simulink subsystem "AUVPlant"  (R2020a)
settings: Solver=VariableStepAuto  StartTime=0.0  StopTime=10.0  RelTol=1e-3
values from neighbouring files (symbols this model uses):
  N = [-39.9215617836 -39.7361560536 -39.4691718024 -38.8907059248 -38.267742672 -37.9562610456 -37.5112872936 -37.2888004176 -36.7993292904 -36.4433502888 -35.8648844112 -35.1974237832 ... (201 elements, 201x1)]    [matlab.mat]    (also in plant_init.m = T200Spec16V{:,6})
  PWM = [1100 1104 1108 1112 1116 1120 1124 1128 1132 1136 1140 1144 ... (201 elements, 201x1)]    [matlab.mat]    (also in plant_init.m = T200Spec16V{:,1})
  tmax = 32    [matlab.mat]
  tmin = -26    [matlab.mat]
undefined symbols (not defined in the file or in its folder): T200
libraries: shared6dof x1, simulink x1, sharedtransform x1
settings Model: Creator=Lamarre  LastModifiedBy=Lamarre

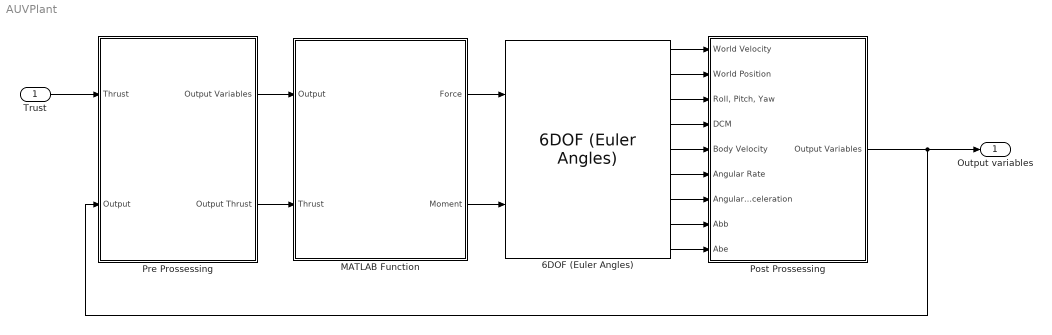
== system AUVPlant ==
  Trust : Inport
  6DOF (Euler Angles) : shared6dof/6DOF (Euler Angles)  units=Metric (MKS)  mtype=Fixed  rep=Quaternion  xme_0=[0 0 0]  Vm_0=[0 0 0]  eul_0=[0 0 0]  pm_0=[0 0 0]  mass_0=mass  mass_e=0.5  mass_f=2.0  inertia=I  inertia_e=eye(3)  inertia_f=2*eye(3)  k_quat=1.0  vre_flag=on  abi_flag=on  aMode=0  xme_statename=''  Vm_statename=''  eul_statename=''  quat_statename=''  pm_statename=''  mass_statename=''
      settings: SourceProductBaseCode=AE,PW,MT,VE,VP
  MATLAB Function : MATLAB Function  TreatAsAtomicUnit=on
  Post Prossessing : Subsystem
  Pre Prossessing : Subsystem
  Output variables : Outport
  wires:
  6DOF (Euler Angles)/4 -> Post Prossessing/4(DCM)
  MATLAB Function/2(Moment) -> 6DOF (Euler Angles)/2
  6DOF (Euler Angles)/6 -> Post Prossessing/6(Angular Rate)
  6DOF (Euler Angles)/5 -> Post Prossessing/5(Body Velocity)
  6DOF (Euler Angles)/2 -> Post Prossessing/2(World Position)
  6DOF (Euler Angles)/1 -> Post Prossessing/1(World Velocity)
  6DOF (Euler Angles)/7 -> Post Prossessing/7(Angular Acceleration)
  MATLAB Function/1(Force) -> 6DOF (Euler Angles)/1
  Post Prossessing/1(Output Variables) -> Output variables/1, Pre Prossessing/2("Output ")
  6DOF (Euler Angles)/3 -> Post Prossessing/3("Roll, Pitch, Yaw")
  Trust/1 -> Pre Prossessing/1(Thrust)
  Pre Prossessing/2(Output Thrust) -> MATLAB Function/2(Thrust)
  Pre Prossessing/1(Output Variables) -> MATLAB Function/1(Output)
  6DOF (Euler Angles)/8 -> Post Prossessing/8(Abb)
  6DOF (Euler Angles)/9 -> Post Prossessing/9(Abe)

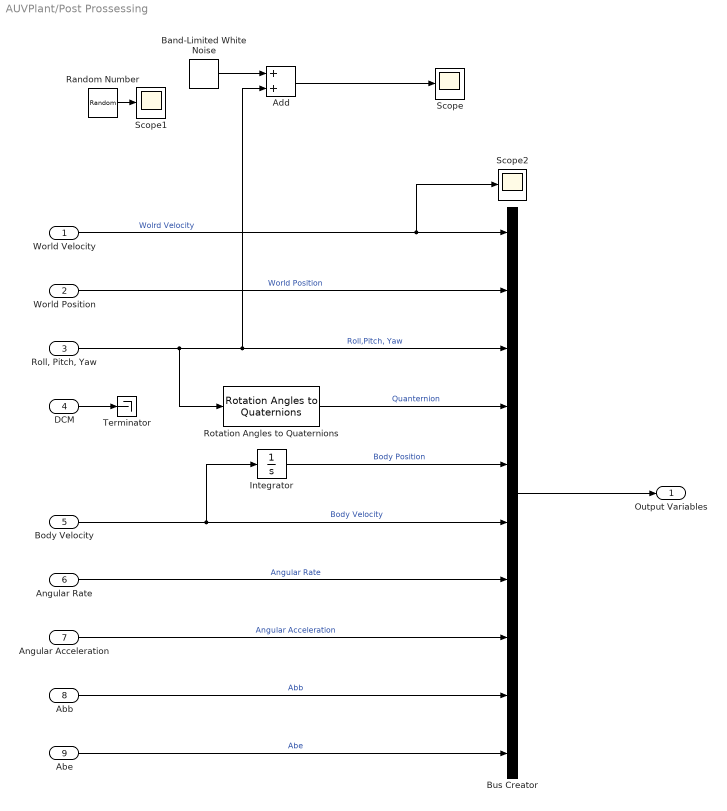
== system AUVPlant/Post Prossessing ==
  World Velocity : Inport
  World Position : Inport  Port=2
  "Roll, Pitch, Yaw" : Inport  Port=3
  DCM : Inport  Port=4
  Body Velocity : Inport  Port=5
  Angular Rate : Inport  Port=6
  Angular Acceleration : Inport  Port=7
  Abb : Inport  Port=8
  Abe : Inport  Port=9
  Add : Sum
  Band-Limited White Noise : simulink/Sources/Band-Limited White Noise  Cov=[0.000000087266]  Ts=1/60  seed=[11111]
  Bus Creator : BusCreator  Inputs=10
  Integrator : Integrator
  Random Number : RandomNumber  Variance=0.0008726  SampleTime=0.01
  Rotation Angles to Quaternions : sharedtransform/Rotation Angles to Quaternions  rotationOrder=XYZ  aMode=aMode
      settings: SourceProductBaseCode=AE,PW,MT,VE,VP
  Scope : Scope
  Scope1 : Scope
  Scope2 : Scope
  Terminator : Terminator
  Output Variables : Outport
  wires:
  DCM/1 -> Terminator/1
  Rotation Angles to Quaternions/1 -> Bus Creator/4  "Quanternion"
  Body Velocity/1 -> Integrator/1, Bus Creator/6  "Body Velocity"
  World Velocity/1 -> Scope2/1, Bus Creator/1  "Wolrd Velocity"
  World Position/1 -> Bus Creator/2  "World Position"
  "Roll, Pitch, Yaw"/1 -> Rotation Angles to Quaternions/1, Add/2, Bus Creator/3  "Roll,Pitch, Yaw"
  Angular Rate/1 -> Bus Creator/7  "Angular Rate"
  Angular Acceleration/1 -> Bus Creator/8  "Angular Acceleration"
  Abb/1 -> Bus Creator/9  "Abb"
  Abe/1 -> Bus Creator/10  "Abe"
  Bus Creator/1 -> Output Variables/1
  Integrator/1 -> Bus Creator/5  "Body Position"
  Band-Limited White Noise/1 -> Add/1
  Add/1 -> Scope/1
  Random Number/1 -> Scope1/1

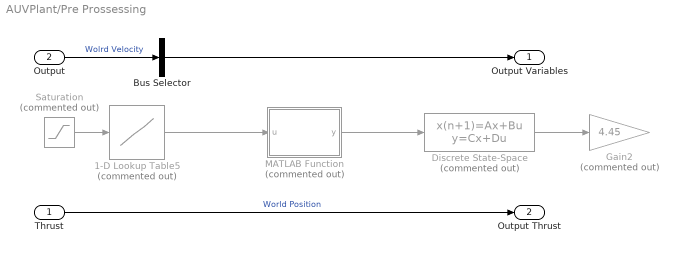
== system AUVPlant/Pre Prossessing ==
  Thrust : Inport
  "Output " : Inport  Port=2
  1-D Lookup Table5 : Lookup_n-D  Commented=on  NumberOfTableDimensions=1  BreakpointsForDimension1=N  Table=PWM  InternalRulePriority=Speed  RndMeth=Simplest  InputSameDT=on
  Bus Selector : BusSelector  OutputSignals=Body Position,Roll;Pitch; Yaw,Body Velocity,Angular Rate  OutputAsBus=on
  Discrete State-Space : DiscreteStateSpace  Commented=on  A=T200.A  B=T200.B  C=T200.C  D=T200.D  SampleTime=T200.Ts
  Gain2 : Gain  Commented=on  Gain=4.45
  MATLAB Function : MATLAB Function  Commented=on  TreatAsAtomicUnit=on
  Saturation : Saturate  Commented=on  UpperLimit=tmax  LowerLimit=tmin  LinearizeAsGain=off  ZeroCross=off
  Output Variables : Outport
  Output Thrust : Outport  Port=2
  wires:
  Thrust/1 -> Output Thrust/1  "World Position"
  Saturation/1 -> 1-D Lookup Table5/1
  1-D Lookup Table5/1 -> MATLAB Function/1(u)
  Discrete State-Space/1 -> Gain2/1
  MATLAB Function/1(y) -> Discrete State-Space/1
  "Output "/1 -> Bus Selector/1  "Wolrd Velocity"
  Bus Selector/1 -> Output Variables/1

== matlab function AUVPlant/MATLAB Function ==
  data: Output input; Force output; Thrust input; Moment output
function [Force,Moment] = Calculate_Forces_and_Torques(Output,Thrust)
Dynamics=AUVForceMoments(Output,Thrust);
Force=Dynamics(1:3);
Moment= Dynamics(4:6);

== matlab function AUVPlant/Pre Prossessing/MATLAB Function ==
  data: u input; y output
function y = fcn(u)
pwm=u-1500;
if pwm>=0 
    y=pwm;
else
   y=pwm*0.77969348659;
end
